simulink model "Mech366Lab1"  (R2024a)
settings: Solver=VariableStepAuto  StartTime=0.0  StopTime=10  RelTol=1e-3
model workspace (MAT data in the model file):
  M1 = Simulink.Parameter
  M1.Value = 1
  M1.Complexity = 'real'
  M1.Dimensions = [1 1]
  M1.DataType = 'auto'
undefined symbols (not defined in the file): F, g, k, M2, mu
settings Model: Creator=luckybhatti  LastModifiedBy=Yoru
settings OptimizationCC: ReuseModelBlockBuffer=off
settings RTWCC: GPUComputeCapability=3.5

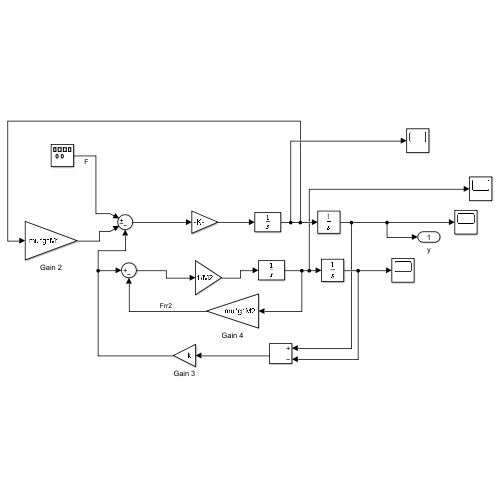
[thumbnail: Simulink's stored preview of the top-level diagram]
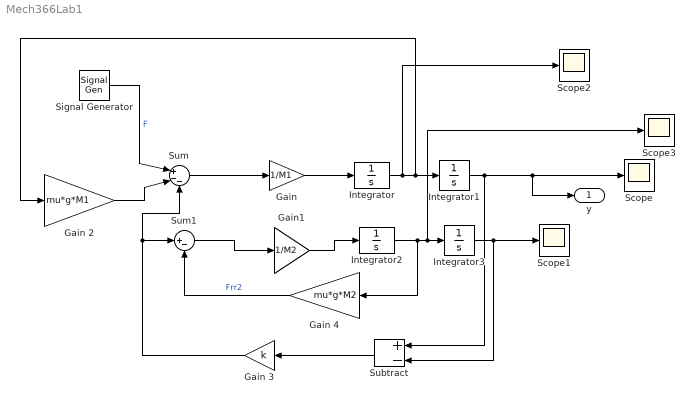
== system Mech366Lab1 ==
  Gain : Gain  Gain=1/M1
  Gain 2 : Gain  Gain=mu*g*M1
  Gain 3 : Gain  Gain=k
  Gain 4 : Gain  Gain=mu*g*M2
  Gain1 : Gain  Gain=1/M2
  Integrator{,1..3} (4 alike) : Integrator
  Scope{,1..3} (4 alike) : Scope
  Signal Generator : SignalGenerator  WaveForm=square  Amplitude=-1*F  Frequency=0.01  Units=rad/sec
  Subtract : Sum  Inputs=+-
  Sum : Sum  Inputs=|+--
  Sum1 : Sum  Inputs=|+-
  y : Outport
  wires:
  Sum/1 -> Gain/1
  Gain/1 -> Integrator/1
  Integrator/1 -> Scope2/1, Gain 2/1, Integrator1/1
  Integrator1/1 -> y/1, Scope/1, Subtract/1
  Integrator3/1 -> Scope1/1, Subtract/2
  Sum1/1 -> Gain1/1
  Gain1/1 -> Integrator2/1
  Integrator2/1 -> Scope3/1, Integrator3/1, Gain 4/1
  Gain 2/1 -> Sum/2
  Signal Generator/1 -> Sum/1  "F"
  Subtract/1 -> Gain 3/1
  Gain 3/1 -> Sum1/1, Sum/3
  Gain 4/1 -> Sum1/2  "Frr2"
